simulink model "project2"  (R2018b)
settings: Solver=VariableStepAuto  StartTime=0.0  StopTime=3  RelTol=1e-3
values from neighbouring files (symbols this model uses):
  a = [a,b]    [lab11.m]
  b = ghg(i)    [LAB5a.m]    (also in lab11.m = a(:, end))
  d = (.01)*(s)*(v.^2)+(.95/s)*((w./v).^2)    [Lab12.m]    (also in lab6_a.m = x(1,1)*x(1,2))
undefined symbols (not defined in the file or in its folder): fc, vo, xo
settings Model: Creator=chris  LastModifiedBy=chris

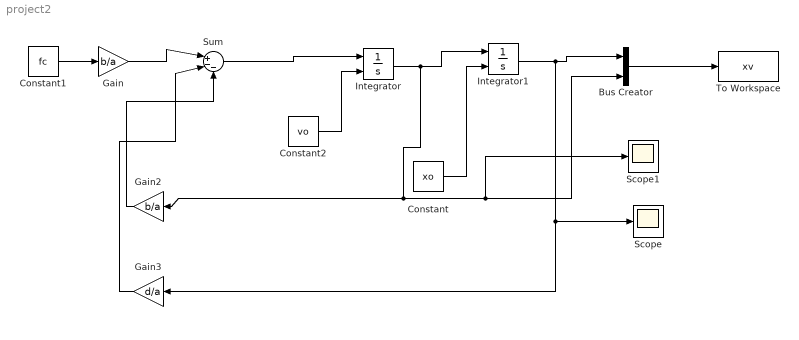
== system project2 ==
  Bus Creator : BusCreator  Inputs=2
  Constant : Constant  Value=xo
  Constant1 : Constant  Value=fc
  Constant2 : Constant  Value=vo
  Gain : Gain  Gain=b/a
  Gain2 : Gain  Gain=b/a
  Gain3 : Gain  Gain=d/a
  Integrator : Integrator  InitialConditionSource=external
  Integrator1 : Integrator  InitialConditionSource=external
  Scope : Scope
  Scope1 : Scope
  Sum : Sum  Inputs=|+--
  To Workspace : ToWorkspace  VariableName=xv  SaveFormat=Timeseries  SampleTime=-1
  wires:
  Constant1/1 -> Gain/1
  Gain/1 -> Sum/1
  Gain3/1 -> Sum/2
  Gain2/1 -> Sum/3
  Sum/1 -> Integrator/1
  Constant2/1 -> Integrator/2
  Integrator/1 -> Gain2/1, Scope1/1, Bus Creator/2, Integrator1/1
  Constant/1 -> Integrator1/2
  Integrator1/1 -> Gain3/1, Scope/1, Bus Creator/1
  Bus Creator/1 -> To Workspace/1
